simulink model "maze_line_path_simulation_new"  (R2020a)
settings: Solver=FixedStepAuto  StartTime=0.0  StopTime=48.4  FixedStep=0.01  RelTol=1e-3  EnableMultiTasking=on
PreLoadFcn:
  | robotParameters_maze;
values from neighbouring files (symbols this model uses):
  axleLength = 0.0672    [robotParameters_maze.m]
  J = 0.0001    [robotParameters_maze.m]
  Kb = 0.190    (= 0.19)    [robotParameters_maze.m]
  Kf = 0.000025    (= 2.5e-05)    [robotParameters_maze.m]
  Km = 0.084    [robotParameters_maze.m]
  L = 0.5    [robotParameters_maze.m]
  mapForSim =     [maze_map.mat]    (also in oval_line_map.mat)
  motorIP = [-12 -11.9 -11.8 -11.7 -11.6 -11.5 -11.4 -11.3 -11.2 -11.1 -11 -10.9 ... (241 elements, 1x241)]    [motorLUT.mat]
  motorSP = [-62.7865560716 -62.2538153955 -61.7309054619 -61.2077148683 -60.684548166 -60.1613790322 -59.6382101464 -59.1150412352 -58.5918723266 -58.0687034178 -57.545534509 -57.0223656001 ... (241 elements, 1x241)]    [motorLUT.mat]
  R = 16    [robotParameters_maze.m]
  wheelR = 0.017    [robotParameters_maze.m]
undefined symbols (not defined in the file or in its folder): DiscIntNeverNeededParam, lineLength
libraries: simulink x6, mobileRoboticsTrainingLib x2, sldrtlib x1
(part 1 of 2)
settings Model: Creator=RAJENDRA PHUTANE  LastModifiedBy=RAJENDRA PHUTANE
settings SolverCC: AutoInsertRateTranBlk=on

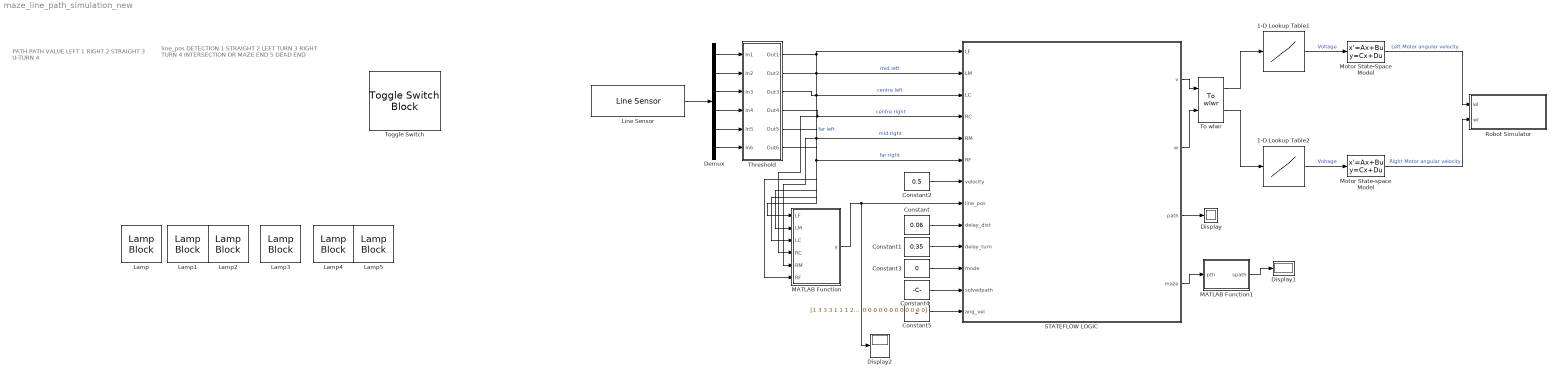
== system maze_line_path_simulation_new ==
  note: PATH
      | PATH VALUE
      |
      | LEFT
      | 1
      |
      | RIGHT
      | 2
      |
      | STRAIGHT
      | 3
      |
      | U-TURN
      | 4
  note: line_pos
      | DETECTION
      |
      | 1
      | STRAIGHT
      |
      | 2
      | LEFT TURN
      |
      | 3
      | RIGHT TURN
      |
      | 4
      | INTERSECTION OR MAZE END
      |
      | 5
      | DEAD END
  1-D Lookup Table1 : Lookup_n-D  NumberOfTableDimensions=1  BreakpointsForDimension1=motorSP  Table=motorIP  ExtrapMethod=Clip  InternalRulePriority=Speed  RndMeth=Simplest  InputSameDT=on
  1-D Lookup Table2 : Lookup_n-D  NumberOfTableDimensions=1  BreakpointsForDimension1=motorSP  Table=motorIP  ExtrapMethod=Clip  InternalRulePriority=Speed  RndMeth=Simplest  InputSameDT=on
  Constant : Constant  Value=0.06
  Constant1 : Constant  Value=0.35
  Constant2 : Constant  Value=0.5
  Constant3 : Constant  Value=0
  Constant4 : Constant  Value="[1 3 3 3 1 1 1 2  0 0 0 0 0 0 0 0 0 0 0 0]"  OutDataTypeStr=single
  Constant5 : Constant  Value=2
  Demux : Demux  Outputs=6
  Display : Display
  Display1 : Display
  Display2 : Display
  Lamp{,1..5} (6 alike) : LampBlock
  Line Sensor : mobileRoboticsTrainingLib/Line Sensor  mapVariable=mapForSim  envVal=0  lineVal=1000  sensOff=[0.075 0.045;0.075 0.027;0.075 0.009;0.075 -0.009;0.075 -0.027;0.075 -0.045]
      settings: SourceProductName=Mobile Robotics Training Library
  MATLAB Function : MATLAB Function  TreatAsAtomicUnit=on
  MATLAB Function1 : MATLAB Function  TreatAsAtomicUnit=on
  Motor State-Space Model : StateSpace  A=[-Kf/J Km/J; -Kb/L -R/L]  B=[0; 1/L]  C=[1 0]  D=[0]  InitialCondition=0
  Motor State-space Model : StateSpace  A=[-Kf/J Km/J; -Kb/L -R/L]  B=[0; 1/L]  C=[1 0]  D=[0]  InitialCondition=0
  Robot Simulator : Subsystem  Priority=99  mask(Robot Simulator){mapVar=mapForSim, startX=0.43994, startY=0.11086, startTheta=90, axleLength=axleLength, wheelR=wheelR}
      mask prompts: mapVar "Map Variable"; startX "Start X (m)"; startY "Start Y (m)"; startTheta "Theta (deg)"; axleLength "Axle Length (m)"; wheelR "Wheel Radius (m)"
      mask help: Configure robot simulator to use custom simulation maps and simulate closed-loop mobile robotics systems along with appropriate sensor simulation blocks.
      mask init:
      | set_param(bdroot,'SolverType','Fixed-Step');
      | set_param(bdroot,'Solver','FixedStepAuto');
      | 
      | if (exist('Ts'))
      |     set_param(bdroot,'FixedStep','Ts');
      | else
      |     set_param(bdroot,'FixedStep','0.01');
      | end
      | h = findobj('Name','Robot Simulator');
      | if ~isempty(h)
      |     close (h);
      | end
      | setupRobotSim();
      mask Help: web('Robot Simulator.htm')
      mask DialogControl mapCont Prompt: Map Setup
      mask DialogControl initPosCont Prompt: Initial Position
      mask DialogControl setPos Prompt: Set position interactively
      mask DialogControl setPos Callback:
      | %% Set starting point
      | setStartingPoint();
      mask DialogControl initOrientation Prompt: Initial Orientation
      mask DialogControl robotCharCont Prompt: Robot Characteristics
      mask Display: disp('Robot Simulator')
  STATEFLOW LOGIC : Stateflow chart  TreatAsAtomicUnit=on
  Threshold : Subsystem
  To wlwr : mobileRoboticsTrainingLib/To wlwr  axleLength=axleLength  wheelR=wheelR
  Toggle Switch : ToggleSwitchBlock  LabelPosition=Hide
      settings: Values={{'Dry Run', 'Shortest Run'}, [0 1]}
  wires:
  STATEFLOW LOGIC/3(path) -> Display/1
  STATEFLOW LOGIC/4(maze) -> MATLAB Function1/1(pth)
  Demux/4 -> Threshold/4(In4)
  1-D Lookup Table1/1 -> Motor State-Space Model/1  "Voltage"
  Constant4/1 -> STATEFLOW LOGIC/12(solvedpath)
  MATLAB Function/1(y) -> Display2/1, STATEFLOW LOGIC/8(line_pos)
  Motor State-space Model/1 -> Robot Simulator/2(wr)  "Right Motor angular velocity"
  Constant3/1 -> STATEFLOW LOGIC/11(mode)
  MATLAB Function1/1(spath) -> Display1/1
  To wlwr/2 -> 1-D Lookup Table2/1
  Motor State-Space Model/1 -> Robot Simulator/1(wl)  "Left Motor angular velocity"
  To wlwr/1 -> 1-D Lookup Table1/1
  Demux/2 -> Threshold/2(In2)
  1-D Lookup Table2/1 -> Motor State-space Model/1  "Voltage"
  Constant1/1 -> STATEFLOW LOGIC/10(delay_turn)
  Constant/1 -> STATEFLOW LOGIC/9(delay_dist)
  STATEFLOW LOGIC/2(w) -> To wlwr/2
  STATEFLOW LOGIC/1(v) -> To wlwr/1
  Constant2/1 -> STATEFLOW LOGIC/7(velocity)
  Demux/3 -> Threshold/3(In3)
  Demux/1 -> Threshold/1(In1)
  Demux/5 -> Threshold/5(In5)
  Demux/6 -> Threshold/6(In6)
  Threshold/1(Out1) -> STATEFLOW LOGIC/1(LF), MATLAB Function/1(LF)  "far left"
  Threshold/5(Out5) -> MATLAB Function/5(RM), STATEFLOW LOGIC/5(RM)  "mid right"
  Threshold/4(Out4) -> MATLAB Function/4(RC), STATEFLOW LOGIC/4(RC)  "centre right"
  Threshold/2(Out2) -> STATEFLOW LOGIC/2(LM), MATLAB Function/2(LM)  "mid left"
  Threshold/3(Out3) -> MATLAB Function/3(LC), STATEFLOW LOGIC/3(LC)  "centre left"
  Threshold/6(Out6) -> MATLAB Function/6(RF), STATEFLOW LOGIC/6(RF)  "far right"
  Line Sensor/1 -> Demux/1
  Constant5/1 -> STATEFLOW LOGIC/13(ang_vel)

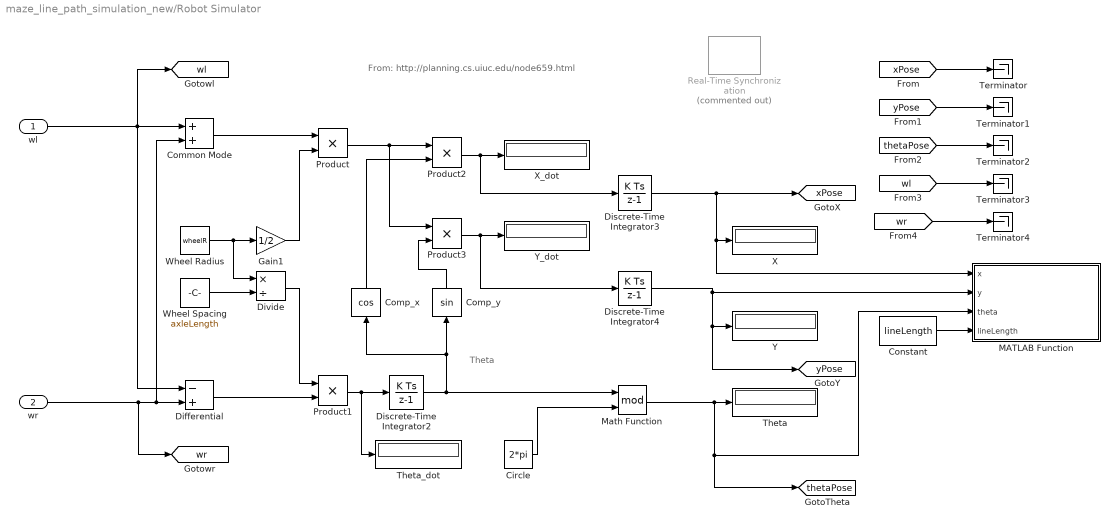
== system maze_line_path_simulation_new/Robot Simulator ==
  note: Theta
  note: From: http://planning.cs.uiuc.edu/node659.html
  wl : Inport
  wr : Inport  Port=2
  Circle : Constant  Value=2*pi
  Common Mode : Sum
  Comp_x : Trigonometry  Operator=cos
  Comp_y : Trigonometry
  Constant : Constant  Value=lineLength
  Differential : Sum  Inputs=-+
  Discrete-Time Integrator2 : DiscreteIntegrator  InitialCondition=startTheta*(pi/180)  SampleTime=-1  ICPrevOutput=DiscIntNeverNeededParam  ICPrevScaledInput=DiscIntNeverNeededParam
  Discrete-Time Integrator3 : DiscreteIntegrator  InitialCondition=startX  SampleTime=-1  ICPrevOutput=DiscIntNeverNeededParam  ICPrevScaledInput=DiscIntNeverNeededParam
  Discrete-Time Integrator4 : DiscreteIntegrator  InitialCondition=startY  SampleTime=-1  ICPrevOutput=DiscIntNeverNeededParam  ICPrevScaledInput=DiscIntNeverNeededParam
  Divide : Product  Inputs=*/
  Gain1 : Gain  Gain=1/2
  MATLAB Function : MATLAB Function  TreatAsAtomicUnit=on
  Math Function : Math  Operator=mod  SignedPower=on  SaturateOnIntegerOverflow=on
  Product{,1..3} (4 alike) : Product  RndMeth=Zero
  Real-Time Synchronization : sldrtlib/Real-Time Synchronization  Commented=on  SampleTime=0.01  MaxMissedTicks=1000  ShowMissedTicks=off  YieldWhenWaiting=off
  Terminator{,1..4} (5 alike) : Terminator
  Theta : Display
  Theta_dot : Display
  Wheel Radius : Constant  Value=wheelR
  Wheel Spacing : Constant  Value=axleLength
  X : Display
  X_dot : Display
  Y : Display
  Y_dot : Display
  tag scope: thetaPose=global, wl=global, wr=global, xPose=global, yPose=global
  wires:
  [wr] -> Terminator4/1
  [wl] -> Terminator3/1
  Math Function/1 -> [thetaPose], MATLAB Function/3(theta), Theta/1
  Differential/1 -> Product1/2
  Comp_y/1 -> Product3/2
  Discrete-Time Integrator3/1 -> [xPose], MATLAB Function/1(x), X/1
  Product3/1 -> Discrete-Time Integrator4/1, Y_dot/1
  Discrete-Time Integrator4/1 -> Y/1, [yPose], MATLAB Function/2(y)
  Divide/1 -> Product1/1
  wr/1 -> [wr], Common Mode/2, Differential/2
  Discrete-Time Integrator2/1 -> Math Function/1, Comp_x/1, Comp_y/1
  wl/1 -> [wl], Common Mode/1, Differential/1
  Comp_x/1 -> Product2/2
  Product1/1 -> Discrete-Time Integrator2/1, Theta_dot/1
  Wheel Radius/1 -> Divide/1, Gain1/1
  Wheel Spacing/1 -> Divide/2
  Product2/1 -> Discrete-Time Integrator3/1, X_dot/1
  Gain1/1 -> Product/2
  Common Mode/1 -> Product/1
  Product/1 -> Product3/1, Product2/1
  Circle/1 -> Math Function/2
  Constant/1 -> MATLAB Function/4(lineLength)
  [xPose] -> Terminator/1
  [yPose] -> Terminator1/1
  [thetaPose] -> Terminator2/1

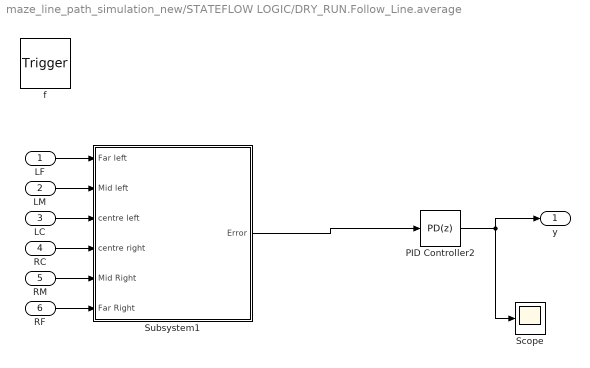
== system maze_line_path_simulation_new/STATEFLOW LOGIC/DRY_RUN.Follow_Line.average ==
  LF : Inport  OutDataTypeStr=double  PortDimensions=1
  LM : Inport  Port=2  OutDataTypeStr=double  PortDimensions=1
  LC : Inport  Port=3  OutDataTypeStr=double  PortDimensions=1
  RC : Inport  Port=4  OutDataTypeStr=double  PortDimensions=1
  RM : Inport  Port=5  OutDataTypeStr=double  PortDimensions=1
  RF : Inport  Port=6  OutDataTypeStr=double  PortDimensions=1
  f : TriggerPort  TriggerType=function-call  VariantControl=(inherit)
      settings: CopyFcn=Stateflow.SLINSF.SimulinkMan.removeBlockPreDeleteFcn  PreDeleteFcn=Stateflow.SLINSF.SimulinkMan.unsafePredeleteFcn
  PID Controller2 : simulink/Continuous/PID Controller  Controller=PD  Form=Parallel  TimeDomain=Discrete-time  UseExternalTs=off  SampleTime=-1  IntegratorMethod=Forward Euler  FilterMethod=Forward Euler  ControllerParametersSource=internal  P=0.9  I=1  D=0.2  UseFilter=on  N=100  TunerSelectOption=Transfer Function Based (PID Tuner App)  InitialConditionSource=internal  InitialConditionForIntegrator=0  InitialConditionForFilter=0  DifferentiatorICPrevScaledInput=0  ExternalReset=none  TrackingMode=off  Kt=1  LimitOutput=off  UpperSaturationLimit=inf  LowerSaturationLimit=-inf  LinearizeAsGain=on  AntiWindupMode=none  Kb=1  POutMin=[]  POutMax=[]  IOutMin=[]  IOutMax=[]  DOutMin=[]  DOutMax=[]  NOutMin=[]  NOutMax=[]  SumOutMin=[]  SumOutMax=[]  SaturationOutMin=[]  SaturationOutMax=[]  PParamMin=[]  PParamMax=[]  IParamMin=[]  IParamMax=[]  DParamMin=[]  DParamMax=[]  NParamMin=[]  NParamMax=[]  KbParamMin=[]  KbParamMax=[]  KtParamMin=[]  KtParamMax=[]  KbOutMin=[]  KbOutMax=[]  KtOutMin=[]  KtOutMax=[]  IntegratorOutMin=[]  IntegratorOutMax=[]  FilterOutMin=[]  FilterOutMax=[]  SumI1OutMin=[]  SumI1OutMax=[]  SumI2OutMin=[]  SumI2OutMax=[]  SumI3OutMin=[]  SumI3OutMax=[]  SumI4OutMin=[]  SumI4OutMax=[]  SumDOutMin=[]  SumDOutMax=[]  DifferentiatorOutMin=[]  DifferentiatorOutMax=[]  FilterDiffOutCoefMin=[]  FilterDiffOutCoefMax=[]  ReciprocalOutMin=[]  ReciprocalOutMax=[]  SumDenOutMin=[]  SumDenOutMax=[]  SumNumOutMin=[]  SumNumOutMax=[]  DivideOutMin=[]  DivideOutMax=[]  UdiffTsProdOutMin=[]  UdiffTsProdOutMax=[]  NTsProdOutMin=[]  NTsProdOutMax=[]  UintegralTsProdOutMin=[]  UintegralTsProdOutMax=[]  UngainTsProdOutMin=[]  UngainTsProdOutMax=[]  IntegratorContinuousStateAttributes=''  IntegratorStateMustResolveToSignalObject=off  IntegratorRTWStateStorageClass=Auto  FilterContinuousStateAttributes=''  FilterStateMustResolveToSignalObject=off  FilterRTWStateStorageClass=Auto  ParallelPVariant=InternalParameters  IdealPVariant=Disabled  IVariant=Disabled  DVariant=InternalParameters  IntegratorVariant=Disabled  SatVariant=Disabled  AWVariant=Disabled  PCopyVariant=Disabled  TRVariant=Disabled  FdbkBlocksVariant=Forward  IdealPFdbkVariant=Disabled  SatFdbkVariant=Disabled  DerivativeFilterVariant=ForwardEulerFilter  NVariant=InternalParameters  NCopyVariant=Disabled  FilterICVariant=InternalICsFilter  IntegratorICVariant=Disabled  ExternalResetVariant=Disabled  TRSumVariant=Passthrough  SumFdbkVariant=Disabled  SumVariant=Sum_PD  TsampFilterVariant=InternalTs  TsampNgainVariant=Passthrough  TsampIntegralVariant=Disabled_SignalSpec  InitialConditionSetting=Output
  Scope : Scope
  Subsystem1 : Subsystem
  y : Outport
  wires:
  PID Controller2/1 -> Scope/1, y/1
  LF/1 -> Subsystem1/1(Far left)
  LM/1 -> Subsystem1/2(Mid left)
  LC/1 -> Subsystem1/3(centre left)
  RC/1 -> Subsystem1/4(centre right)
  RM/1 -> Subsystem1/5(Mid Right)
  RF/1 -> Subsystem1/6(Far Right)
  Subsystem1/1(Error) -> PID Controller2/1

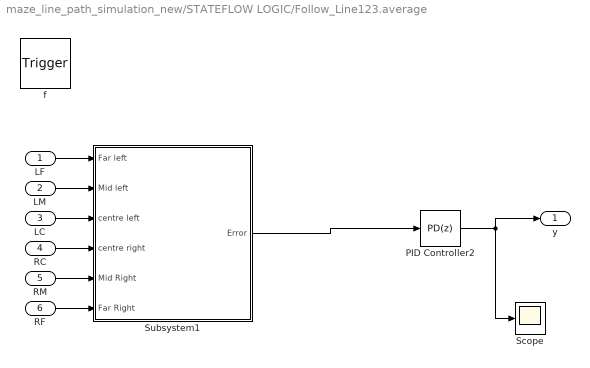
== system maze_line_path_simulation_new/STATEFLOW LOGIC/Follow_Line123.average ==
  LF : Inport  OutDataTypeStr=double  PortDimensions=1
  LM : Inport  Port=2  OutDataTypeStr=double  PortDimensions=1
  LC : Inport  Port=3  OutDataTypeStr=double  PortDimensions=1
  RC : Inport  Port=4  OutDataTypeStr=double  PortDimensions=1
  RM : Inport  Port=5  OutDataTypeStr=double  PortDimensions=1
  RF : Inport  Port=6  OutDataTypeStr=double  PortDimensions=1
  f : TriggerPort  TriggerType=function-call  VariantControl=(inherit)
      settings: CopyFcn=Stateflow.SLINSF.SimulinkMan.removeBlockPreDeleteFcn  PreDeleteFcn=Stateflow.SLINSF.SimulinkMan.unsafePredeleteFcn
  PID Controller2 : simulink/Continuous/PID Controller  Controller=PD  Form=Parallel  TimeDomain=Discrete-time  UseExternalTs=off  SampleTime=-1  IntegratorMethod=Forward Euler  FilterMethod=Forward Euler  ControllerParametersSource=internal  P=2  I=1  D=1e-4  UseFilter=on  N=100  TunerSelectOption=Transfer Function Based (PID Tuner App)  InitialConditionSource=internal  InitialConditionForIntegrator=0  InitialConditionForFilter=0  DifferentiatorICPrevScaledInput=0  ExternalReset=none  TrackingMode=off  Kt=1  LimitOutput=off  UpperSaturationLimit=inf  LowerSaturationLimit=-inf  LinearizeAsGain=on  AntiWindupMode=none  Kb=1  POutMin=[]  POutMax=[]  IOutMin=[]  IOutMax=[]  DOutMin=[]  DOutMax=[]  NOutMin=[]  NOutMax=[]  SumOutMin=[]  SumOutMax=[]  SaturationOutMin=[]  SaturationOutMax=[]  PParamMin=[]  PParamMax=[]  IParamMin=[]  IParamMax=[]  DParamMin=[]  DParamMax=[]  NParamMin=[]  NParamMax=[]  KbParamMin=[]  KbParamMax=[]  KtParamMin=[]  KtParamMax=[]  KbOutMin=[]  KbOutMax=[]  KtOutMin=[]  KtOutMax=[]  IntegratorOutMin=[]  IntegratorOutMax=[]  FilterOutMin=[]  FilterOutMax=[]  SumI1OutMin=[]  SumI1OutMax=[]  SumI2OutMin=[]  SumI2OutMax=[]  SumI3OutMin=[]  SumI3OutMax=[]  SumI4OutMin=[]  SumI4OutMax=[]  SumDOutMin=[]  SumDOutMax=[]  DifferentiatorOutMin=[]  DifferentiatorOutMax=[]  FilterDiffOutCoefMin=[]  FilterDiffOutCoefMax=[]  ReciprocalOutMin=[]  ReciprocalOutMax=[]  SumDenOutMin=[]  SumDenOutMax=[]  SumNumOutMin=[]  SumNumOutMax=[]  DivideOutMin=[]  DivideOutMax=[]  UdiffTsProdOutMin=[]  UdiffTsProdOutMax=[]  NTsProdOutMin=[]  NTsProdOutMax=[]  UintegralTsProdOutMin=[]  UintegralTsProdOutMax=[]  UngainTsProdOutMin=[]  UngainTsProdOutMax=[]  IntegratorContinuousStateAttributes=''  IntegratorStateMustResolveToSignalObject=off  IntegratorRTWStateStorageClass=Auto  FilterContinuousStateAttributes=''  FilterStateMustResolveToSignalObject=off  FilterRTWStateStorageClass=Auto  ParallelPVariant=InternalParameters  IdealPVariant=Disabled  IVariant=Disabled  DVariant=InternalParameters  IntegratorVariant=Disabled  SatVariant=Disabled  AWVariant=Disabled  PCopyVariant=Disabled  TRVariant=Disabled  FdbkBlocksVariant=Forward  IdealPFdbkVariant=Disabled  SatFdbkVariant=Disabled  DerivativeFilterVariant=ForwardEulerFilter  NVariant=InternalParameters  NCopyVariant=Disabled  FilterICVariant=InternalICsFilter  IntegratorICVariant=Disabled  ExternalResetVariant=Disabled  TRSumVariant=Passthrough  SumFdbkVariant=Disabled  SumVariant=Sum_PD  TsampFilterVariant=InternalTs  TsampNgainVariant=Passthrough  TsampIntegralVariant=Disabled_SignalSpec  InitialConditionSetting=Output
  Scope : Scope
  Subsystem1 : Subsystem
  y : Outport
  wires:
  PID Controller2/1 -> Scope/1, y/1
  LF/1 -> Subsystem1/1(Far left)
  LM/1 -> Subsystem1/2(Mid left)
  LC/1 -> Subsystem1/3(centre left)
  RC/1 -> Subsystem1/4(centre right)
  RM/1 -> Subsystem1/5(Mid Right)
  RF/1 -> Subsystem1/6(Far Right)
  Subsystem1/1(Error) -> PID Controller2/1

== system maze_line_path_simulation_new/STATEFLOW LOGIC/Follow_Line14.average ==
  LF : Inport  OutDataTypeStr=double  PortDimensions=1
  LM : Inport  Port=2  OutDataTypeStr=double  PortDimensions=1
  LC : Inport  Port=3  OutDataTypeStr=double  PortDimensions=1
  RC : Inport  Port=4  OutDataTypeStr=double  PortDimensions=1
  RM : Inport  Port=5  OutDataTypeStr=double  PortDimensions=1
  RF : Inport  Port=6  OutDataTypeStr=double  PortDimensions=1
  f : TriggerPort  TriggerType=function-call  VariantControl=(inherit)
      settings: CopyFcn=Stateflow.SLINSF.SimulinkMan.removeBlockPreDeleteFcn  PreDeleteFcn=Stateflow.SLINSF.SimulinkMan.unsafePredeleteFcn
  PID Controller2 : simulink/Continuous/PID Controller  Controller=PD  Form=Parallel  TimeDomain=Discrete-time  UseExternalTs=off  SampleTime=-1  IntegratorMethod=Forward Euler  FilterMethod=Forward Euler  ControllerParametersSource=internal  P=2  I=1  D=1e-4  UseFilter=on  N=100  TunerSelectOption=Transfer Function Based (PID Tuner App)  InitialConditionSource=internal  InitialConditionForIntegrator=0  InitialConditionForFilter=0  DifferentiatorICPrevScaledInput=0  ExternalReset=none  TrackingMode=off  Kt=1  LimitOutput=off  UpperSaturationLimit=inf  LowerSaturationLimit=-inf  LinearizeAsGain=on  AntiWindupMode=none  Kb=1  POutMin=[]  POutMax=[]  IOutMin=[]  IOutMax=[]  DOutMin=[]  DOutMax=[]  NOutMin=[]  NOutMax=[]  SumOutMin=[]  SumOutMax=[]  SaturationOutMin=[]  SaturationOutMax=[]  PParamMin=[]  PParamMax=[]  IParamMin=[]  IParamMax=[]  DParamMin=[]  DParamMax=[]  NParamMin=[]  NParamMax=[]  KbParamMin=[]  KbParamMax=[]  KtParamMin=[]  KtParamMax=[]  KbOutMin=[]  KbOutMax=[]  KtOutMin=[]  KtOutMax=[]  IntegratorOutMin=[]  IntegratorOutMax=[]  FilterOutMin=[]  FilterOutMax=[]  SumI1OutMin=[]  SumI1OutMax=[]  SumI2OutMin=[]  SumI2OutMax=[]  SumI3OutMin=[]  SumI3OutMax=[]  SumI4OutMin=[]  SumI4OutMax=[]  SumDOutMin=[]  SumDOutMax=[]  DifferentiatorOutMin=[]  DifferentiatorOutMax=[]  FilterDiffOutCoefMin=[]  FilterDiffOutCoefMax=[]  ReciprocalOutMin=[]  ReciprocalOutMax=[]  SumDenOutMin=[]  SumDenOutMax=[]  SumNumOutMin=[]  SumNumOutMax=[]  DivideOutMin=[]  DivideOutMax=[]  UdiffTsProdOutMin=[]  UdiffTsProdOutMax=[]  NTsProdOutMin=[]  NTsProdOutMax=[]  UintegralTsProdOutMin=[]  UintegralTsProdOutMax=[]  UngainTsProdOutMin=[]  UngainTsProdOutMax=[]  IntegratorContinuousStateAttributes=''  IntegratorStateMustResolveToSignalObject=off  IntegratorRTWStateStorageClass=Auto  FilterContinuousStateAttributes=''  FilterStateMustResolveToSignalObject=off  FilterRTWStateStorageClass=Auto  ParallelPVariant=InternalParameters  IdealPVariant=Disabled  IVariant=Disabled  DVariant=InternalParameters  IntegratorVariant=Disabled  SatVariant=Disabled  AWVariant=Disabled  PCopyVariant=Disabled  TRVariant=Disabled  FdbkBlocksVariant=Forward  IdealPFdbkVariant=Disabled  SatFdbkVariant=Disabled  DerivativeFilterVariant=ForwardEulerFilter  NVariant=InternalParameters  NCopyVariant=Disabled  FilterICVariant=InternalICsFilter  IntegratorICVariant=Disabled  ExternalResetVariant=Disabled  TRSumVariant=Passthrough  SumFdbkVariant=Disabled  SumVariant=Sum_PD  TsampFilterVariant=InternalTs  TsampNgainVariant=Passthrough  TsampIntegralVariant=Disabled_SignalSpec  InitialConditionSetting=Output
  Scope : Scope
  Subsystem1 : Subsystem
  y : Outport
  wires:
  PID Controller2/1 -> Scope/1, y/1
  LF/1 -> Subsystem1/1(Far left)
  LM/1 -> Subsystem1/2(Mid left)
  LC/1 -> Subsystem1/3(centre left)
  RC/1 -> Subsystem1/4(centre right)
  RM/1 -> Subsystem1/5(Mid Right)
  RF/1 -> Subsystem1/6(Far Right)
  Subsystem1/1(Error) -> PID Controller2/1

== system maze_line_path_simulation_new/STATEFLOW LOGIC/Follow_Line2.average ==
  LF : Inport  OutDataTypeStr=double  PortDimensions=1
  LM : Inport  Port=2  OutDataTypeStr=double  PortDimensions=1
  LC : Inport  Port=3  OutDataTypeStr=double  PortDimensions=1
  RC : Inport  Port=4  OutDataTypeStr=double  PortDimensions=1
  RM : Inport  Port=5  OutDataTypeStr=double  PortDimensions=1
  RF : Inport  Port=6  OutDataTypeStr=double  PortDimensions=1
  f : TriggerPort  TriggerType=function-call  VariantControl=(inherit)
      settings: CopyFcn=Stateflow.SLINSF.SimulinkMan.removeBlockPreDeleteFcn  PreDeleteFcn=Stateflow.SLINSF.SimulinkMan.unsafePredeleteFcn
  PID Controller2 : simulink/Continuous/PID Controller  Controller=PD  Form=Parallel  TimeDomain=Discrete-time  UseExternalTs=off  SampleTime=-1  IntegratorMethod=Forward Euler  FilterMethod=Forward Euler  ControllerParametersSource=internal  P=2  I=1  D=1e-4  UseFilter=on  N=100  TunerSelectOption=Transfer Function Based (PID Tuner App)  InitialConditionSource=internal  InitialConditionForIntegrator=0  InitialConditionForFilter=0  DifferentiatorICPrevScaledInput=0  ExternalReset=none  TrackingMode=off  Kt=1  LimitOutput=off  UpperSaturationLimit=inf  LowerSaturationLimit=-inf  LinearizeAsGain=on  AntiWindupMode=none  Kb=1  POutMin=[]  POutMax=[]  IOutMin=[]  IOutMax=[]  DOutMin=[]  DOutMax=[]  NOutMin=[]  NOutMax=[]  SumOutMin=[]  SumOutMax=[]  SaturationOutMin=[]  SaturationOutMax=[]  PParamMin=[]  PParamMax=[]  IParamMin=[]  IParamMax=[]  DParamMin=[]  DParamMax=[]  NParamMin=[]  NParamMax=[]  KbParamMin=[]  KbParamMax=[]  KtParamMin=[]  KtParamMax=[]  KbOutMin=[]  KbOutMax=[]  KtOutMin=[]  KtOutMax=[]  IntegratorOutMin=[]  IntegratorOutMax=[]  FilterOutMin=[]  FilterOutMax=[]  SumI1OutMin=[]  SumI1OutMax=[]  SumI2OutMin=[]  SumI2OutMax=[]  SumI3OutMin=[]  SumI3OutMax=[]  SumI4OutMin=[]  SumI4OutMax=[]  SumDOutMin=[]  SumDOutMax=[]  DifferentiatorOutMin=[]  DifferentiatorOutMax=[]  FilterDiffOutCoefMin=[]  FilterDiffOutCoefMax=[]  ReciprocalOutMin=[]  ReciprocalOutMax=[]  SumDenOutMin=[]  SumDenOutMax=[]  SumNumOutMin=[]  SumNumOutMax=[]  DivideOutMin=[]  DivideOutMax=[]  UdiffTsProdOutMin=[]  UdiffTsProdOutMax=[]  NTsProdOutMin=[]  NTsProdOutMax=[]  UintegralTsProdOutMin=[]  UintegralTsProdOutMax=[]  UngainTsProdOutMin=[]  UngainTsProdOutMax=[]  IntegratorContinuousStateAttributes=''  IntegratorStateMustResolveToSignalObject=off  IntegratorRTWStateStorageClass=Auto  FilterContinuousStateAttributes=''  FilterStateMustResolveToSignalObject=off  FilterRTWStateStorageClass=Auto  ParallelPVariant=InternalParameters  IdealPVariant=Disabled  IVariant=Disabled  DVariant=InternalParameters  IntegratorVariant=Disabled  SatVariant=Disabled  AWVariant=Disabled  PCopyVariant=Disabled  TRVariant=Disabled  FdbkBlocksVariant=Forward  IdealPFdbkVariant=Disabled  SatFdbkVariant=Disabled  DerivativeFilterVariant=ForwardEulerFilter  NVariant=InternalParameters  NCopyVariant=Disabled  FilterICVariant=InternalICsFilter  IntegratorICVariant=Disabled  ExternalResetVariant=Disabled  TRSumVariant=Passthrough  SumFdbkVariant=Disabled  SumVariant=Sum_PD  TsampFilterVariant=InternalTs  TsampNgainVariant=Passthrough  TsampIntegralVariant=Disabled_SignalSpec  InitialConditionSetting=Output
  Scope : Scope
  Subsystem1 : Subsystem
  y : Outport
  wires:
  PID Controller2/1 -> Scope/1, y/1
  LF/1 -> Subsystem1/1(Far left)
  LM/1 -> Subsystem1/2(Mid left)
  LC/1 -> Subsystem1/3(centre left)
  RC/1 -> Subsystem1/4(centre right)
  RM/1 -> Subsystem1/5(Mid Right)
  RF/1 -> Subsystem1/6(Far Right)
  Subsystem1/1(Error) -> PID Controller2/1

== system maze_line_path_simulation_new/STATEFLOW LOGIC/Follow_Line32.average ==
  LF : Inport  OutDataTypeStr=double  PortDimensions=1
  LM : Inport  Port=2  OutDataTypeStr=double  PortDimensions=1
  LC : Inport  Port=3  OutDataTypeStr=double  PortDimensions=1
  RC : Inport  Port=4  OutDataTypeStr=double  PortDimensions=1
  RM : Inport  Port=5  OutDataTypeStr=double  PortDimensions=1
  RF : Inport  Port=6  OutDataTypeStr=double  PortDimensions=1
  f : TriggerPort  TriggerType=function-call  VariantControl=(inherit)
      settings: CopyFcn=Stateflow.SLINSF.SimulinkMan.removeBlockPreDeleteFcn  PreDeleteFcn=Stateflow.SLINSF.SimulinkMan.unsafePredeleteFcn
  PID Controller2 : simulink/Continuous/PID Controller  Controller=PD  Form=Parallel  TimeDomain=Discrete-time  UseExternalTs=off  SampleTime=-1  IntegratorMethod=Forward Euler  FilterMethod=Forward Euler  ControllerParametersSource=internal  P=2  I=1  D=1e-4  UseFilter=on  N=100  TunerSelectOption=Transfer Function Based (PID Tuner App)  InitialConditionSource=internal  InitialConditionForIntegrator=0  InitialConditionForFilter=0  DifferentiatorICPrevScaledInput=0  ExternalReset=none  TrackingMode=off  Kt=1  LimitOutput=off  UpperSaturationLimit=inf  LowerSaturationLimit=-inf  LinearizeAsGain=on  AntiWindupMode=none  Kb=1  POutMin=[]  POutMax=[]  IOutMin=[]  IOutMax=[]  DOutMin=[]  DOutMax=[]  NOutMin=[]  NOutMax=[]  SumOutMin=[]  SumOutMax=[]  SaturationOutMin=[]  SaturationOutMax=[]  PParamMin=[]  PParamMax=[]  IParamMin=[]  IParamMax=[]  DParamMin=[]  DParamMax=[]  NParamMin=[]  NParamMax=[]  KbParamMin=[]  KbParamMax=[]  KtParamMin=[]  KtParamMax=[]  KbOutMin=[]  KbOutMax=[]  KtOutMin=[]  KtOutMax=[]  IntegratorOutMin=[]  IntegratorOutMax=[]  FilterOutMin=[]  FilterOutMax=[]  SumI1OutMin=[]  SumI1OutMax=[]  SumI2OutMin=[]  SumI2OutMax=[]  SumI3OutMin=[]  SumI3OutMax=[]  SumI4OutMin=[]  SumI4OutMax=[]  SumDOutMin=[]  SumDOutMax=[]  DifferentiatorOutMin=[]  DifferentiatorOutMax=[]  FilterDiffOutCoefMin=[]  FilterDiffOutCoefMax=[]  ReciprocalOutMin=[]  ReciprocalOutMax=[]  SumDenOutMin=[]  SumDenOutMax=[]  SumNumOutMin=[]  SumNumOutMax=[]  DivideOutMin=[]  DivideOutMax=[]  UdiffTsProdOutMin=[]  UdiffTsProdOutMax=[]  NTsProdOutMin=[]  NTsProdOutMax=[]  UintegralTsProdOutMin=[]  UintegralTsProdOutMax=[]  UngainTsProdOutMin=[]  UngainTsProdOutMax=[]  IntegratorContinuousStateAttributes=''  IntegratorStateMustResolveToSignalObject=off  IntegratorRTWStateStorageClass=Auto  FilterContinuousStateAttributes=''  FilterStateMustResolveToSignalObject=off  FilterRTWStateStorageClass=Auto  ParallelPVariant=InternalParameters  IdealPVariant=Disabled  IVariant=Disabled  DVariant=InternalParameters  IntegratorVariant=Disabled  SatVariant=Disabled  AWVariant=Disabled  PCopyVariant=Disabled  TRVariant=Disabled  FdbkBlocksVariant=Forward  IdealPFdbkVariant=Disabled  SatFdbkVariant=Disabled  DerivativeFilterVariant=ForwardEulerFilter  NVariant=InternalParameters  NCopyVariant=Disabled  FilterICVariant=InternalICsFilter  IntegratorICVariant=Disabled  ExternalResetVariant=Disabled  TRSumVariant=Passthrough  SumFdbkVariant=Disabled  SumVariant=Sum_PD  TsampFilterVariant=InternalTs  TsampNgainVariant=Passthrough  TsampIntegralVariant=Disabled_SignalSpec  InitialConditionSetting=Output
  Scope : Scope
  Subsystem1 : Subsystem
  y : Outport
  wires:
  PID Controller2/1 -> Scope/1, y/1
  LF/1 -> Subsystem1/1(Far left)
  LM/1 -> Subsystem1/2(Mid left)
  LC/1 -> Subsystem1/3(centre left)
  RC/1 -> Subsystem1/4(centre right)
  RM/1 -> Subsystem1/5(Mid Right)
  RF/1 -> Subsystem1/6(Far Right)
  Subsystem1/1(Error) -> PID Controller2/1

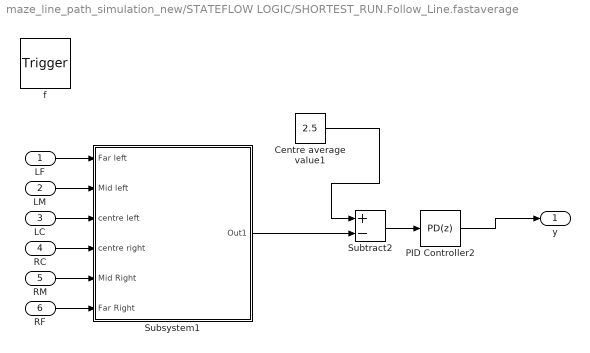
== system maze_line_path_simulation_new/STATEFLOW LOGIC/SHORTEST_RUN.Follow_Line.fastaverage ==
  LF : Inport  OutDataTypeStr=double  PortDimensions=1
  LM : Inport  Port=2  OutDataTypeStr=double  PortDimensions=1
  LC : Inport  Port=3  OutDataTypeStr=double  PortDimensions=1
  RC : Inport  Port=4  OutDataTypeStr=double  PortDimensions=1
  RM : Inport  Port=5  OutDataTypeStr=double  PortDimensions=1
  RF : Inport  Port=6  OutDataTypeStr=double  PortDimensions=1
  f : TriggerPort  TriggerType=function-call  VariantControl=(inherit)
      settings: CopyFcn=Stateflow.SLINSF.SimulinkMan.removeBlockPreDeleteFcn  PreDeleteFcn=Stateflow.SLINSF.SimulinkMan.unsafePredeleteFcn
  Centre average value1 : Constant  Value=2.5
  PID Controller2 : simulink/Continuous/PID Controller  Controller=PD  Form=Parallel  TimeDomain=Discrete-time  UseExternalTs=off  SampleTime=-1  IntegratorMethod=Forward Euler  FilterMethod=Forward Euler  ControllerParametersSource=internal  P=1.2  I=1  D=0.1  UseFilter=on  N=100  TunerSelectOption=Transfer Function Based (PID Tuner App)  InitialConditionSource=internal  InitialConditionForIntegrator=0  InitialConditionForFilter=0  DifferentiatorICPrevScaledInput=0  ExternalReset=none  TrackingMode=off  Kt=1  LimitOutput=off  UpperSaturationLimit=inf  LowerSaturationLimit=-inf  LinearizeAsGain=on  AntiWindupMode=none  Kb=1  POutMin=[]  POutMax=[]  IOutMin=[]  IOutMax=[]  DOutMin=[]  DOutMax=[]  NOutMin=[]  NOutMax=[]  SumOutMin=[]  SumOutMax=[]  SaturationOutMin=[]  SaturationOutMax=[]  PParamMin=[]  PParamMax=[]  IParamMin=[]  IParamMax=[]  DParamMin=[]  DParamMax=[]  NParamMin=[]  NParamMax=[]  KbParamMin=[]  KbParamMax=[]  KtParamMin=[]  KtParamMax=[]  KbOutMin=[]  KbOutMax=[]  KtOutMin=[]  KtOutMax=[]  IntegratorOutMin=[]  IntegratorOutMax=[]  FilterOutMin=[]  FilterOutMax=[]  SumI1OutMin=[]  SumI1OutMax=[]  SumI2OutMin=[]  SumI2OutMax=[]  SumI3OutMin=[]  SumI3OutMax=[]  SumI4OutMin=[]  SumI4OutMax=[]  SumDOutMin=[]  SumDOutMax=[]  DifferentiatorOutMin=[]  DifferentiatorOutMax=[]  FilterDiffOutCoefMin=[]  FilterDiffOutCoefMax=[]  ReciprocalOutMin=[]  ReciprocalOutMax=[]  SumDenOutMin=[]  SumDenOutMax=[]  SumNumOutMin=[]  SumNumOutMax=[]  DivideOutMin=[]  DivideOutMax=[]  UdiffTsProdOutMin=[]  UdiffTsProdOutMax=[]  NTsProdOutMin=[]  NTsProdOutMax=[]  UintegralTsProdOutMin=[]  UintegralTsProdOutMax=[]  UngainTsProdOutMin=[]  UngainTsProdOutMax=[]  IntegratorContinuousStateAttributes=''  IntegratorStateMustResolveToSignalObject=off  IntegratorRTWStateStorageClass=Auto  FilterContinuousStateAttributes=''  FilterStateMustResolveToSignalObject=off  FilterRTWStateStorageClass=Auto  ParallelPVariant=InternalParameters  IdealPVariant=Disabled  IVariant=Disabled  DVariant=InternalParameters  IntegratorVariant=Disabled  SatVariant=Disabled  AWVariant=Disabled  PCopyVariant=Disabled  TRVariant=Disabled  FdbkBlocksVariant=Forward  IdealPFdbkVariant=Disabled  SatFdbkVariant=Disabled  DerivativeFilterVariant=ForwardEulerFilter  NVariant=InternalParameters  NCopyVariant=Disabled  FilterICVariant=InternalICsFilter  IntegratorICVariant=Disabled  ExternalResetVariant=Disabled  TRSumVariant=Passthrough  SumFdbkVariant=Disabled  SumVariant=Sum_PD  TsampFilterVariant=InternalTs  TsampNgainVariant=Passthrough  TsampIntegralVariant=Disabled_SignalSpec  InitialConditionSetting=Output
  Subsystem1 : Subsystem
  Subtract2 : Sum  Inputs=+-
  y : Outport
  wires:
  Subsystem1/1(Out1) -> Subtract2/2
  Subtract2/1 -> PID Controller2/1
  PID Controller2/1 -> y/1
  Centre average value1/1 -> Subtract2/1
  LF/1 -> Subsystem1/1(Far left)
  LM/1 -> Subsystem1/2(Mid left)
  LC/1 -> Subsystem1/3(centre left)
  RC/1 -> Subsystem1/4(centre right)
  RM/1 -> Subsystem1/5(Mid Right)
  RF/1 -> Subsystem1/6(Far Right)

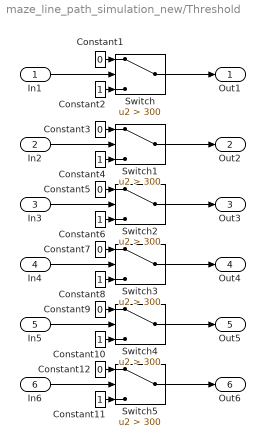
== system maze_line_path_simulation_new/Threshold ==
  In1 : Inport
  In2 : Inport  Port=2
  In3 : Inport  Port=3
  In4 : Inport  Port=4
  In5 : Inport  Port=5
  In6 : Inport  Port=6
  Constant{1,3,5,7,9,12} (6 alike) : Constant  Value=0
  Constant{2,4,6,8,10..11} (6 alike) : Constant
  Switch{,1..5} (6 alike) : Switch  Criteria=u2 > Threshold  Threshold=300
  Out1 : Outport
  Out2 : Outport  Port=2
  Out3 : Outport  Port=3
  Out4 : Outport  Port=4
  Out5 : Outport  Port=5
  Out6 : Outport  Port=6
  wires:
  Constant2/1 -> Switch/3
  Constant1/1 -> Switch/1
  Switch/1 -> Out1/1
  In1/1 -> Switch/2
  In2/1 -> Switch1/2
  Switch1/1 -> Out2/1
  Constant3/1 -> Switch1/1
  Constant4/1 -> Switch1/3
  Constant6/1 -> Switch2/3
  Constant5/1 -> Switch2/1
  Switch2/1 -> Out3/1
  In3/1 -> Switch2/2
  In4/1 -> Switch3/2
  Switch3/1 -> Out4/1
  Constant7/1 -> Switch3/1
  Constant8/1 -> Switch3/3
  Constant10/1 -> Switch4/3
  Constant9/1 -> Switch4/1
  Switch4/1 -> Out5/1
  In5/1 -> Switch4/2
  In6/1 -> Switch5/2
  Switch5/1 -> Out6/1
  Constant12/1 -> Switch5/1
  Constant11/1 -> Switch5/3

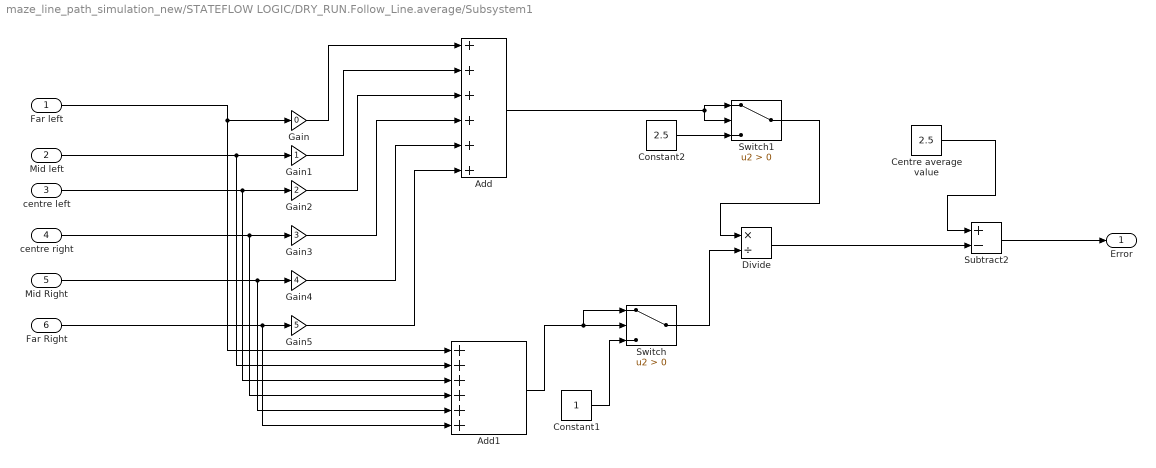
== system maze_line_path_simulation_new/STATEFLOW LOGIC/DRY_RUN.Follow_Line.average/Subsystem1 ==
  Far left : Inport
  Mid left : Inport  Port=2
  centre left : Inport  Port=3
  centre right : Inport  Port=4
  Mid Right : Inport  Port=5
  Far Right : Inport  Port=6
  Add : Sum  Inputs=++++++
  Add1 : Sum  Inputs=++++++
  Centre average value : Constant  Value=2.5
  Constant1 : Constant
  Constant2 : Constant  Value=2.5
  Divide : Product  Inputs=*/
  Gain : Gain  Gain=0
  Gain1 : Gain
  Gain2 : Gain  Gain=2
  Gain3 : Gain  Gain=3
  Gain4 : Gain  Gain=4
  Gain5 : Gain  Gain=5
  Subtract2 : Sum  Inputs=+-
  Switch : Switch  Criteria=u2 > Threshold
  Switch1 : Switch  Criteria=u2 > Threshold
  Error : Outport
  wires:
  Constant2/1 -> Switch1/3
  Mid left/1 -> Gain1/1, Add1/2
  Gain2/1 -> Add/3
  Mid Right/1 -> Gain4/1, Add1/5
  Gain/1 -> Add/1
  Switch/1 -> Divide/2
  Add/1 -> Switch1/2, Switch1/1
  Constant1/1 -> Switch/3
  Add1/1 -> Switch/2, Switch/1
  Gain3/1 -> Add/4
  Gain1/1 -> Add/2
  Gain4/1 -> Add/5
  centre right/1 -> Gain3/1, Add1/4
  Far Right/1 -> Gain5/1, Add1/6
  centre left/1 -> Gain2/1, Add1/3
  Gain5/1 -> Add/6
  Far left/1 -> Gain/1, Add1/1
  Switch1/1 -> Divide/1
  Divide/1 -> Subtract2/2
  Centre average value/1 -> Subtract2/1
  Subtract2/1 -> Error/1

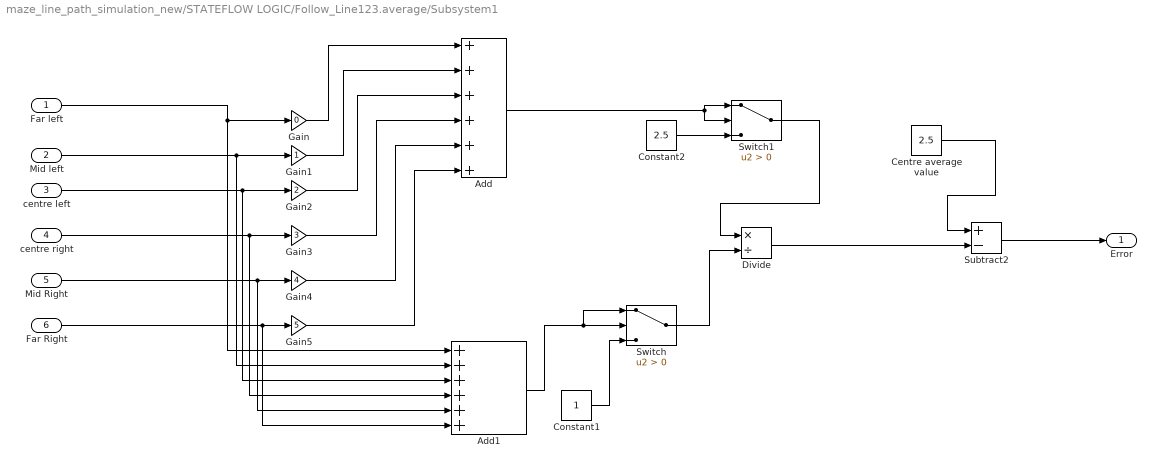
== system maze_line_path_simulation_new/STATEFLOW LOGIC/Follow_Line123.average/Subsystem1 ==
  Far left : Inport
  Mid left : Inport  Port=2
  centre left : Inport  Port=3
  centre right : Inport  Port=4
  Mid Right : Inport  Port=5
  Far Right : Inport  Port=6
  Add : Sum  Inputs=++++++
  Add1 : Sum  Inputs=++++++
  Centre average value : Constant  Value=2.5
  Constant1 : Constant
  Constant2 : Constant  Value=2.5
  Divide : Product  Inputs=*/
  Gain : Gain  Gain=0
  Gain1 : Gain
  Gain2 : Gain  Gain=2
  Gain3 : Gain  Gain=3
  Gain4 : Gain  Gain=4
  Gain5 : Gain  Gain=5
  Subtract2 : Sum  Inputs=+-
  Switch : Switch  Criteria=u2 > Threshold
  Switch1 : Switch  Criteria=u2 > Threshold
  Error : Outport
  wires:
  Constant2/1 -> Switch1/3
  Mid left/1 -> Gain1/1, Add1/2
  Gain2/1 -> Add/3
  Mid Right/1 -> Gain4/1, Add1/5
  Gain/1 -> Add/1
  Switch/1 -> Divide/2
  Add/1 -> Switch1/2, Switch1/1
  Constant1/1 -> Switch/3
  Add1/1 -> Switch/2, Switch/1
  Gain3/1 -> Add/4
  Gain1/1 -> Add/2
  Gain4/1 -> Add/5
  centre right/1 -> Gain3/1, Add1/4
  Far Right/1 -> Gain5/1, Add1/6
  centre left/1 -> Gain2/1, Add1/3
  Gain5/1 -> Add/6
  Far left/1 -> Gain/1, Add1/1
  Switch1/1 -> Divide/1
  Divide/1 -> Subtract2/2
  Centre average value/1 -> Subtract2/1
  Subtract2/1 -> Error/1

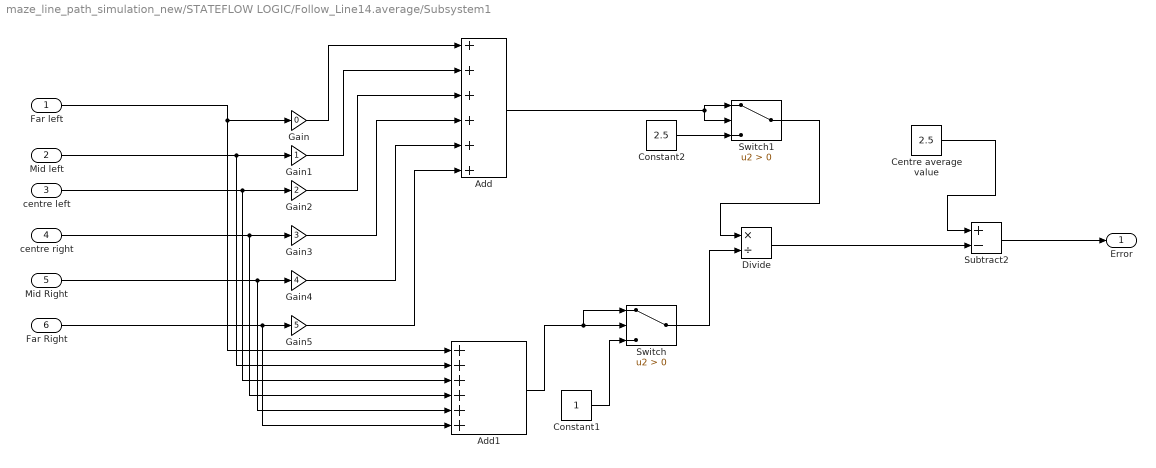
== system maze_line_path_simulation_new/STATEFLOW LOGIC/Follow_Line14.average/Subsystem1 ==
  Far left : Inport
  Mid left : Inport  Port=2
  centre left : Inport  Port=3
  centre right : Inport  Port=4
  Mid Right : Inport  Port=5
  Far Right : Inport  Port=6
  Add : Sum  Inputs=++++++
  Add1 : Sum  Inputs=++++++
  Centre average value : Constant  Value=2.5
  Constant1 : Constant
  Constant2 : Constant  Value=2.5
  Divide : Product  Inputs=*/
  Gain : Gain  Gain=0
  Gain1 : Gain
  Gain2 : Gain  Gain=2
  Gain3 : Gain  Gain=3
  Gain4 : Gain  Gain=4
  Gain5 : Gain  Gain=5
  Subtract2 : Sum  Inputs=+-
  Switch : Switch  Criteria=u2 > Threshold
  Switch1 : Switch  Criteria=u2 > Threshold
  Error : Outport
  wires:
  Constant2/1 -> Switch1/3
  Mid left/1 -> Gain1/1, Add1/2
  Gain2/1 -> Add/3
  Mid Right/1 -> Gain4/1, Add1/5
  Gain/1 -> Add/1
  Switch/1 -> Divide/2
  Add/1 -> Switch1/2, Switch1/1
  Constant1/1 -> Switch/3
  Add1/1 -> Switch/2, Switch/1
  Gain3/1 -> Add/4
  Gain1/1 -> Add/2
  Gain4/1 -> Add/5
  centre right/1 -> Gain3/1, Add1/4
  Far Right/1 -> Gain5/1, Add1/6
  centre left/1 -> Gain2/1, Add1/3
  Gain5/1 -> Add/6
  Far left/1 -> Gain/1, Add1/1
  Switch1/1 -> Divide/1
  Divide/1 -> Subtract2/2
  Centre average value/1 -> Subtract2/1
  Subtract2/1 -> Error/1

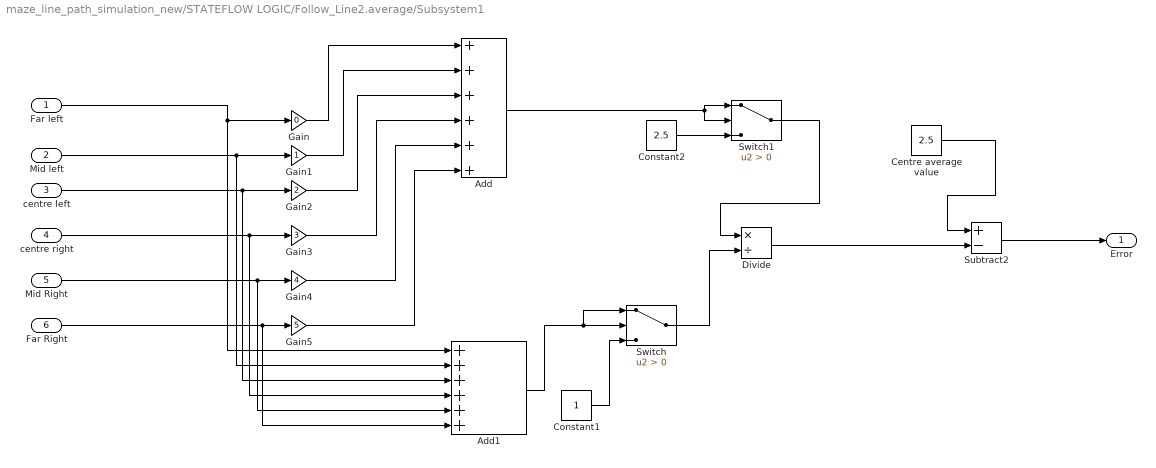
== system maze_line_path_simulation_new/STATEFLOW LOGIC/Follow_Line2.average/Subsystem1 ==
  Far left : Inport
  Mid left : Inport  Port=2
  centre left : Inport  Port=3
  centre right : Inport  Port=4
  Mid Right : Inport  Port=5
  Far Right : Inport  Port=6
  Add : Sum  Inputs=++++++
  Add1 : Sum  Inputs=++++++
  Centre average value : Constant  Value=2.5
  Constant1 : Constant
  Constant2 : Constant  Value=2.5
  Divide : Product  Inputs=*/
  Gain : Gain  Gain=0
  Gain1 : Gain
  Gain2 : Gain  Gain=2
  Gain3 : Gain  Gain=3
  Gain4 : Gain  Gain=4
  Gain5 : Gain  Gain=5
  Subtract2 : Sum  Inputs=+-
  Switch : Switch  Criteria=u2 > Threshold
  Switch1 : Switch  Criteria=u2 > Threshold
  Error : Outport
  wires:
  Constant2/1 -> Switch1/3
  Mid left/1 -> Gain1/1, Add1/2
  Gain2/1 -> Add/3
  Mid Right/1 -> Gain4/1, Add1/5
  Gain/1 -> Add/1
  Switch/1 -> Divide/2
  Add/1 -> Switch1/2, Switch1/1
  Constant1/1 -> Switch/3
  Add1/1 -> Switch/2, Switch/1
  Gain3/1 -> Add/4
  Gain1/1 -> Add/2
  Gain4/1 -> Add/5
  centre right/1 -> Gain3/1, Add1/4
  Far Right/1 -> Gain5/1, Add1/6
  centre left/1 -> Gain2/1, Add1/3
  Gain5/1 -> Add/6
  Far left/1 -> Gain/1, Add1/1
  Switch1/1 -> Divide/1
  Divide/1 -> Subtract2/2
  Centre average value/1 -> Subtract2/1
  Subtract2/1 -> Error/1

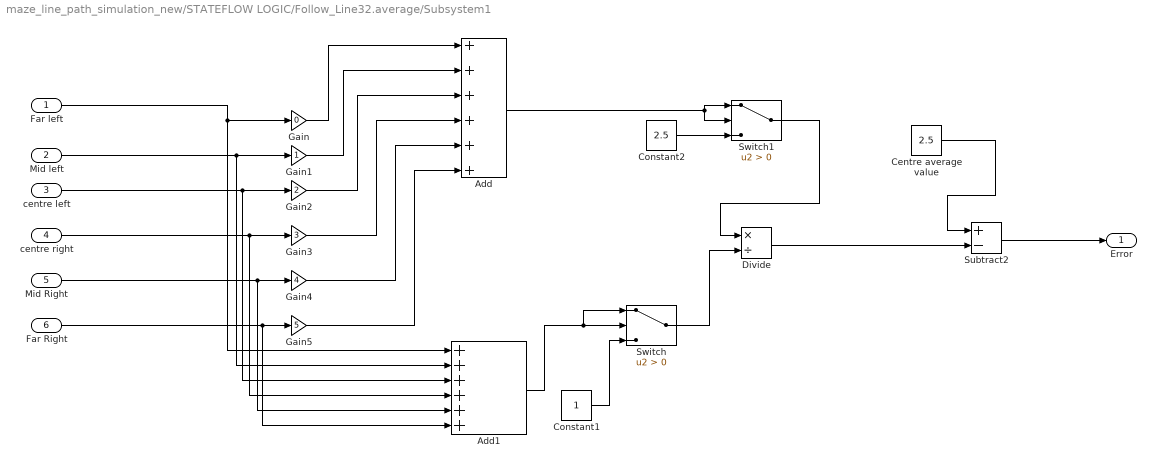
== system maze_line_path_simulation_new/STATEFLOW LOGIC/Follow_Line32.average/Subsystem1 ==
  Far left : Inport
  Mid left : Inport  Port=2
  centre left : Inport  Port=3
  centre right : Inport  Port=4
  Mid Right : Inport  Port=5
  Far Right : Inport  Port=6
  Add : Sum  Inputs=++++++
  Add1 : Sum  Inputs=++++++
  Centre average value : Constant  Value=2.5
  Constant1 : Constant
  Constant2 : Constant  Value=2.5
  Divide : Product  Inputs=*/
  Gain : Gain  Gain=0
  Gain1 : Gain
  Gain2 : Gain  Gain=2
  Gain3 : Gain  Gain=3
  Gain4 : Gain  Gain=4
  Gain5 : Gain  Gain=5
  Subtract2 : Sum  Inputs=+-
  Switch : Switch  Criteria=u2 > Threshold
  Switch1 : Switch  Criteria=u2 > Threshold
  Error : Outport
  wires:
  Constant2/1 -> Switch1/3
  Mid left/1 -> Gain1/1, Add1/2
  Gain2/1 -> Add/3
  Mid Right/1 -> Gain4/1, Add1/5
  Gain/1 -> Add/1
  Switch/1 -> Divide/2
  Add/1 -> Switch1/2, Switch1/1
  Constant1/1 -> Switch/3
  Add1/1 -> Switch/2, Switch/1
  Gain3/1 -> Add/4
  Gain1/1 -> Add/2
  Gain4/1 -> Add/5
  centre right/1 -> Gain3/1, Add1/4
  Far Right/1 -> Gain5/1, Add1/6
  centre left/1 -> Gain2/1, Add1/3
  Gain5/1 -> Add/6
  Far left/1 -> Gain/1, Add1/1
  Switch1/1 -> Divide/1
  Divide/1 -> Subtract2/2
  Centre average value/1 -> Subtract2/1
  Subtract2/1 -> Error/1

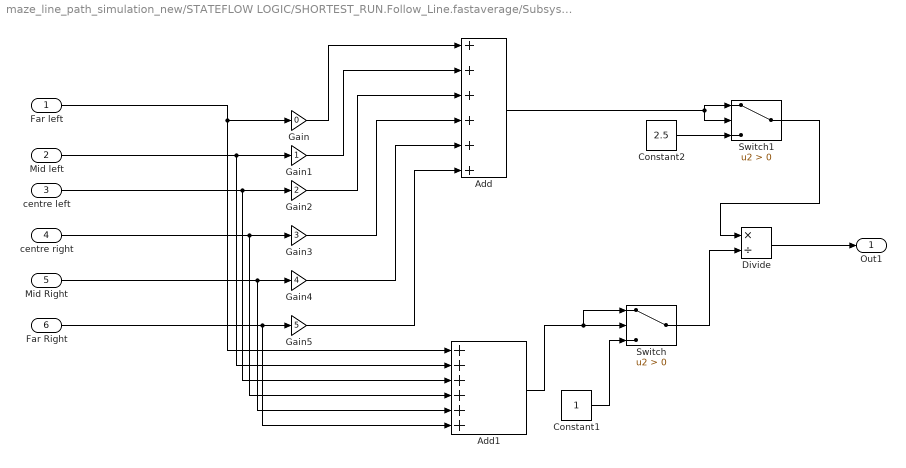
== system maze_line_path_simulation_new/STATEFLOW LOGIC/SHORTEST_RUN.Follow_Line.fastaverage/Subsystem1 ==
  Far left : Inport
  Mid left : Inport  Port=2
  centre left : Inport  Port=3
  centre right : Inport  Port=4
  Mid Right : Inport  Port=5
  Far Right : Inport  Port=6
  Add : Sum  Inputs=++++++
  Add1 : Sum  Inputs=++++++
  Constant1 : Constant
  Constant2 : Constant  Value=2.5
  Divide : Product  Inputs=*/
  Gain : Gain  Gain=0
  Gain1 : Gain
  Gain2 : Gain  Gain=2
  Gain3 : Gain  Gain=3
  Gain4 : Gain  Gain=4
  Gain5 : Gain  Gain=5
  Switch : Switch  Criteria=u2 > Threshold
  Switch1 : Switch  Criteria=u2 > Threshold
  Out1 : Outport
  wires:
  Constant2/1 -> Switch1/3
  Mid left/1 -> Gain1/1, Add1/2
  Gain2/1 -> Add/3
  Mid Right/1 -> Gain4/1, Add1/5
  Gain/1 -> Add/1
  Switch/1 -> Divide/2
  Add/1 -> Switch1/2, Switch1/1
  Constant1/1 -> Switch/3
  Add1/1 -> Switch/2, Switch/1
  Gain3/1 -> Add/4
  Gain1/1 -> Add/2
  Gain4/1 -> Add/5
  centre right/1 -> Gain3/1, Add1/4
  Far Right/1 -> Gain5/1, Add1/6
  centre left/1 -> Gain2/1, Add1/3
  Gain5/1 -> Add/6
  Far left/1 -> Gain/1, Add1/1
  Switch1/1 -> Divide/1
  Divide/1 -> Out1/1

== matlab function maze_line_path_simulation_new/MATLAB Function ==
  data: LF input; y output; LM input; LC input; RC input; RM input; RF input
function y = fcn(LF,LM,LC,RC,RM,RF)
if(LF==0 && LM==0 && LC==1 && RC==1 && RM==0 && RF==0)
    line=1;   % LINE ON CENTRE (001100)
elseif(LF==1 && LM==1 && LC==1 && RC==1 && RM==0 && RF==0)
    line=2;   % LINE ON LEFT (111100)
elseif(LF==0 && LM==0 && LC==1 && RC==1 && RM==1 && RF==1)
    line=3;   % LINE ON RIGHT (001111)
elseif(LF==1 && LM==1 && LC==1 && RC==1 && RM==1 && RF==1)
    line=4;   % INTERSECTION OR END DETECTED (111111)
else(LF==0 && LM==0 && LC==0 && RC==0 && RM==0 && RF==0)
    line=5;   % DEAD END DETECTED (000000)
end
y = line;

== matlab function maze_line_path_simulation_new/MATLAB Function1 ==
  data: pth input; spath output
function spath= trails(pth)
for j=1:5  
 for i=1:20
     if pth(i)==4
         if pth(i-1)==1
           
            if pth(i+1)==1 %______141
             pth(i-1)=3;
             pth(i)=0;
             pth(i+1)=0;
             [~, S] = sort(pth == 0, 2);
            Index  = sub2ind(size(pth), repmat((1:1).', 1, 20), S);
            pth= pth(Index);
           elseif pth(i+1)==2 %____142
             pth(i-1)=4;
             pth(i)=0;
             pth(i+1)=0;
             [~, S] = sort(pth == 0, 2);
             Index  = sub2ind(size(pth), repmat((1:1).', 1, 20), S);
             pth= pth(Index);
           else
             pth(i-1)=2;
             pth(i)=0;
             pth(i+1)=0;
             [~, S] = sort(pth == 0, 2);
             Index  = sub2ind(size(pth), repmat((1:1).', 1, 20), S);
             pth= pth(Index);
            end  
          
         elseif pth(i-1)==2
            if pth(i+1)==1
             pth(i-1)=4;
             pth(i)=0;
             pth(i+1)=0;
               [~, S] = sort(pth == 0, 2);
            Index  = sub2ind(size(pth), repmat((1:1).', 1, 20), S);
            pth= pth(Index);
           elseif pth(i+1)==2 
             pth(i-1)=3;
             pth(i)=0;
             pth(i+1)=0;
               [~, S] = sort(pth == 0, 2);
            Index  = sub2ind(size(pth), repmat((1:1).', 1, 20), S);
            pth= pth(Index);
           else
             pth(i-1)=1;
             pth(i)=0;
             pth(i+1)=0;
               [~, S] = sort(pth == 0, 2);
            Index  = sub2ind(size(pth), repmat((1:1).', 1, 20), S);
            pth= pth(Index);
            end
          
         else
            if pth(i-1)==3 
             if pth(i+1)==1
             pth(i-1)=2;
             pth(i)=0;
             pth(i+1)=0;
               [~, S] = sort(pth == 0, 2);
            Index  = sub2ind(size(pth), repmat((1:1).', 1, 20), S);
            pth= pth(Index);
            elseif pth(i+1)==2
              pth(i-1)=1;
              pth(i)=0;
              pth(i+1)=0;
                [~, S] = sort(pth == 0, 2);
            Index  = sub2ind(size(pth), repmat((1:1).', 1, 20), S);
            pth= pth(Index);
            else
                pth(i-1)=4;
                pth(i)=0;
                pth(i+1)=0;
                  [~, S] = sort(pth == 0, 2);
            Index  = sub2ind(size(pth), repmat((1:1).', 1, 20), S);
            pth= pth(Index);
            end 
            end 
         end  
     end    
        % break;
  end    
 end


spath=pth;
